simulink model "kirchImplementation"  (R2020b)
settings: Solver=VariableStepAuto  StartTime=0.0  StopTime=Ts  RelTol=1e-3
InitFcn:
  | evalin('base','pixelcontrolbus');
  | 
  | ROWS = 480;
  | COLS = 752;
  | 
  | OFFSET = 2;
  | imagesToRead = 20;
  | Ts = imagesToRead + OFFSET;
  | 
  | inputNums = [1:imagesToRead];
  | 
  | NUM_OF_BITS = 32;
  | MSB = NUM_OF_BITS-1;
  | cap_1 = fixdt(0,NUM_OF_BITS,NUM_OF_BITS-1);
  | cap_2 = fixdt(0,NUM_OF_BITS,NUM_OF_BITS-2);
  | 
  | CORDIC_LUT_DT_1 = fixdt(1, NUM_OF_BITS, NUM_OF_BITS-2);
  | CORDIC_LUT_DT_2 = fixdt(1, NUM_OF_BITS, NUM_OF_BITS-1);
  | CORDIC_LUT_DT_3 = fixdt(1, NUM_OF_BITS, NUM_OF_BITS);
  | CORDIC_LUT_DT_4 = fixdt(1, NUM_OF_BITS, NUM_OF_BITS+1);
  | CORDIC_LUT_DT_5 = fixdt(1, NUM_OF_BITS, NUM_OF_BITS+1);
  | CORDIC_LUT_DT_6 = fixdt(1, NUM_OF_BITS, NUM_OF_BITS+2);
  | CORDIC_LUT_DT_7 = fixdt(1, NUM_OF_BITS, NUM_OF_BITS+3);
  | CORDIC_LUT_DT_8 = fixdt(1, NUM_OF_BITS, NUM_OF_BITS+4);
  | CORDIC_LUT_DT_9 = fixdt(1, NUM_OF_BITS, NUM_OF_BITS+5);
  | CORDIC_LUT_DT_10 = fixdt(1, NUM_OF_BITS, NUM_OF_BITS+6);
  | CORDIC_LUT_DT_11 = fixdt(1, NUM_OF_BITS, NUM_OF_BITS+7);
  | CORDIC_LUT_DT_12 = fixdt(1, NUM_OF_BITS, NUM_OF_BITS+8);
  | 
  | RGB_DT = fixdt(0, 24, 0);
  | GRAY_DT = fixdt(0, 8, 0);
  | THETA_DT = fixdt(1, 16, 13);
  | MAG_DT = fixdt(0, 16, 15);
  | KIRCH_DT = fixdt(0, 12, 0);
  | 
  | OUTPUT_SIZE = RGB_DT.WordLength + ...
  |     GRAY_DT.WordLength + ...
  |     THETA_DT.WordLength + ...
  |     MAG_DT.WordLength + ...
  |     KIRCH_DT.WordLength*4;
  | 
  | RGB_MSB = OUTPUT_SIZE;
  | GRAY_MSB = RGB_MSB - RGB_DT.WordLength;
  | THETA_MSB = GRAY_MSB - GRAY_DT.WordLength;
  | MAG_MSB = THETA_MSB - THETA_DT.WordLength;
  | KIRCH_MSB = MAG_MSB - MAG_DT.WordLength;
StopFcn:
  | for i = inputNums
  | %% Get output data
  | 
  | %raw = out.raw.data(:,:,i+OFFSET);
  | rgb = out.RGB.data(:,:,:,i+OFFSET);
  | gray = out.gray.data(:,:,i+OFFSET);
  | theta = out.theta.data(:,:,i+OFFSET);
  | mag = out.mag.data(:,:,i+OFFSET);
  | kirch_north = uint16(out.kirch_north.data(:,:,i+OFFSET));
  | kirch_northwest = uint16(out.kirch_northwest.data(:,:,i+OFFSET));
  | kirch_west = uint16(out.kirch_west.data(:,:,i+OFFSET));
  | kirch_southwest = uint16(out.kirch_southwest.data(:,:,i+OFFSET));
  | 
  | %% Write out raw data
  | 
  | %writematrix(raw, sprintf("./data/raw%d.csv", i));
  | writematrix(rgb, sprintf("./data/rgb%d.csv", i));
  | writematrix(gray, sprintf("./data/gray%d.csv", i));
  | 
  | writematrix(theta, sprintf("./data/theta%d.csv", i));
  | writematrix(mag, sprintf("./data/mag%d.csv", i));
  | 
  | writematrix(kirch_north, sprintf("./data/kirch_north%d.csv", i));
  | writematrix(kirch_northwest, sprintf("./data/kirch_northwest%d.csv", i));
  | writematrix(kirch_west, sprintf("./data/kirch_west%d.csv", i));
  | writematrix(kirch_southwest, sprintf("./data/kirch_southwest%d.csv", i));
  | end
libraries: hdlsllib x69, visionhdlio x10, simulink x2
(part 1 of 2)
settings Model: Creator=tyson  LastModifiedBy=tyson

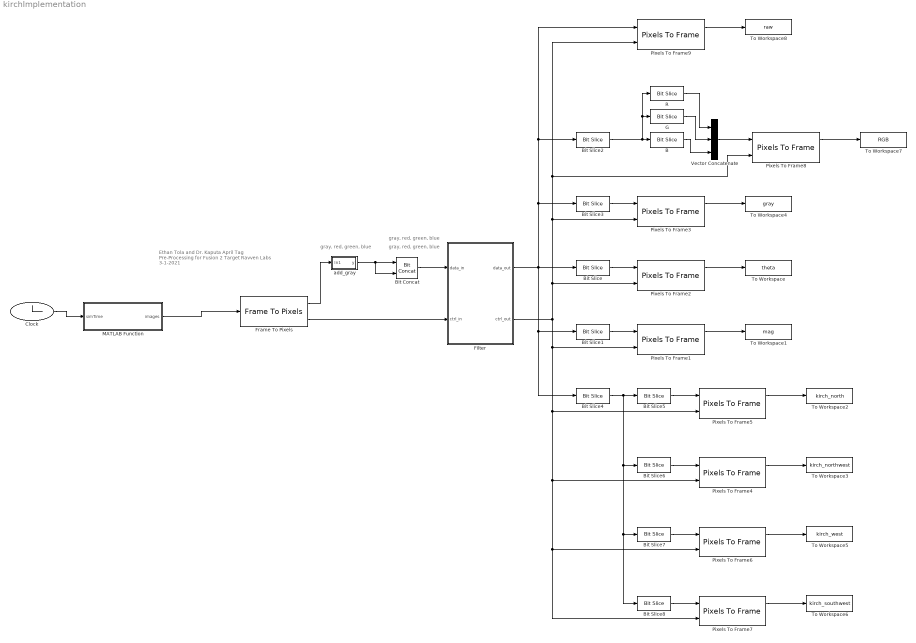
== system kirchImplementation ==
  note: Ethan Tola and Dr. Kaputa
      | April Tag Pre-Processing for Fusion 2 Target
      | Ravven Labs
      | 3-1-2021
  note: gray, red, green, blue
  note: gray, red, green, blue
  note: gray, red, green, blue
  B : hdlsllib/Logic and Bit Operations/Bit Slice  lidx=7  ridx=0
      settings: SourceProductBaseCode=SL
  Bit Concat : hdlsllib/Logic and Bit Operations/Bit Concat  numInputs=2
  Bit Slice : hdlsllib/Logic and Bit Operations/Bit Slice  lidx=THETA_MSB - 1  ridx=THETA_MSB - THETA_DT.WordLength
      settings: SourceProductBaseCode=SL
  Bit Slice1 : hdlsllib/Logic and Bit Operations/Bit Slice  lidx=MAG_MSB - 1  ridx=MAG_MSB - MAG_DT.WordLength
      settings: SourceProductBaseCode=SL
  Bit Slice2 : hdlsllib/Logic and Bit Operations/Bit Slice  lidx=RGB_MSB - 1  ridx=RGB_MSB - RGB_DT.WordLength
      settings: SourceProductBaseCode=SL
  Bit Slice3 : hdlsllib/Logic and Bit Operations/Bit Slice  lidx=GRAY_MSB - 1  ridx=GRAY_MSB - GRAY_DT.WordLength
      settings: SourceProductBaseCode=SL
  Bit Slice4 : hdlsllib/Logic and Bit Operations/Bit Slice  lidx=KIRCH_MSB - 1  ridx=0
      settings: SourceProductBaseCode=SL
  Bit Slice5 : hdlsllib/Logic and Bit Operations/Bit Slice  lidx=KIRCH_MSB - 1  ridx=KIRCH_MSB - KIRCH_DT.WordLength * 1
      settings: SourceProductBaseCode=SL
  Bit Slice6 : hdlsllib/Logic and Bit Operations/Bit Slice  lidx=KIRCH_MSB - (KIRCH_DT.WordLength * 1) - 1  ridx=KIRCH_MSB - KIRCH_DT.WordLength * 2
      settings: SourceProductBaseCode=SL
  Bit Slice7 : hdlsllib/Logic and Bit Operations/Bit Slice  lidx=KIRCH_MSB - (KIRCH_DT.WordLength * 2) - 1  ridx=KIRCH_MSB - KIRCH_DT.WordLength * 3
      settings: SourceProductBaseCode=SL
  Bit Slice8 : hdlsllib/Logic and Bit Operations/Bit Slice  lidx=KIRCH_MSB - (KIRCH_DT.WordLength * 3) - 1  ridx=0
      settings: SourceProductBaseCode=SL
  Clock : Clock
  Filter : Subsystem  TreatAsAtomicUnit=on
  Frame To Pixels : visionhdlio/Frame To Pixels  NumComponents=3  NumPixels=1  VideoFormat=Custom  ActivePixelsPerLine=752  ActiveVideoLines=480  TotalPixelsPerLine=752  TotalVideoLines=480  StartingActiveLine=1  FrontPorch=0  SampleTime=0
      settings: SourceProductName=Vision HDL Toolbox
  G : hdlsllib/Logic and Bit Operations/Bit Slice  lidx=15  ridx=8
      settings: SourceProductBaseCode=SL
  MATLAB Function : MATLAB Function  TreatAsAtomicUnit=on  SystemSampleTime=1
  Pixels To Frame{1..7,9} (8 alike) : visionhdlio/Pixels To Frame  NumComponents=1  NumPixels=1  VideoFormat=Custom  ActivePixelsPerLine=752  ActiveVideoLines=480  TotalPixelsPerLine=752  TotalVideoLines=480
      settings: SourceProductBaseCode=VT
  Pixels To Frame8 : visionhdlio/Pixels To Frame  NumComponents=3  NumPixels=1  VideoFormat=Custom  ActivePixelsPerLine=752  ActiveVideoLines=480  TotalPixelsPerLine=752  TotalVideoLines=480
      settings: SourceProductBaseCode=VT
  R : hdlsllib/Logic and Bit Operations/Bit Slice  lidx=23  ridx=16
      settings: SourceProductBaseCode=SL
  To Workspace : ToWorkspace  VariableName=theta  SaveFormat=Timeseries  SampleTime=-1
  To Workspace1 : ToWorkspace  VariableName=mag  SaveFormat=Timeseries  SampleTime=-1
  To Workspace2 : ToWorkspace  VariableName=kirch_north  SaveFormat=Timeseries  SampleTime=-1
  To Workspace3 : ToWorkspace  VariableName=kirch_northwest  SaveFormat=Timeseries  SampleTime=-1
  To Workspace4 : ToWorkspace  VariableName=gray  SaveFormat=Timeseries  SampleTime=-1
  To Workspace5 : ToWorkspace  VariableName=kirch_west  SaveFormat=Timeseries  SampleTime=-1
  To Workspace6 : ToWorkspace  VariableName=kirch_southwest  SaveFormat=Timeseries  SampleTime=-1
  To Workspace7 : ToWorkspace  VariableName=RGB  SaveFormat=Timeseries  SampleTime=-1
  To Workspace8 : ToWorkspace  VariableName=raw  SaveFormat=Timeseries  SampleTime=-1
  Vector Concatenate : Concatenate  NumInputs=3  Mode=Multidimensional array  ConcatenateDimension=2
  add_gray : Subsystem
  wires:
  Frame To Pixels/1 -> add_gray/1(In1)
  Bit Concat/1 -> Filter/1(data_in)
  Bit Slice1/1 -> Pixels To Frame1/1
  Bit Slice/1 -> Pixels To Frame2/1
  Pixels To Frame2/1 -> To Workspace/1
  Filter/1(data_out) -> Pixels To Frame9/1, Bit Slice2/1, Bit Slice3/1, Bit Slice/1, Bit Slice4/1, Bit Slice1/1
  Pixels To Frame1/1 -> To Workspace1/1
  add_gray/1(y) -> Bit Concat/2, Bit Concat/1
  Filter/2(ctrl_out) -> Pixels To Frame9/2, Pixels To Frame8/2, Pixels To Frame3/2, Pixels To Frame2/2, Pixels To Frame7/2, Pixels To Frame6/2, Pixels To Frame4/2, Pixels To Frame5/2, Pixels To Frame1/2
  Frame To Pixels/2 -> Filter/2(ctrl_in)
  Pixels To Frame7/1 -> To Workspace6/1
  Pixels To Frame5/1 -> To Workspace2/1
  Pixels To Frame4/1 -> To Workspace3/1
  Pixels To Frame6/1 -> To Workspace5/1
  Pixels To Frame3/1 -> To Workspace4/1
  Pixels To Frame8/1 -> To Workspace7/1
  Bit Slice3/1 -> Pixels To Frame3/1
  Bit Slice8/1 -> Pixels To Frame7/1
  Bit Slice7/1 -> Pixels To Frame6/1
  Bit Slice6/1 -> Pixels To Frame4/1
  Bit Slice5/1 -> Pixels To Frame5/1
  Bit Slice4/1 -> Bit Slice8/1, Bit Slice7/1, Bit Slice6/1, Bit Slice5/1
  R/1 -> Vector Concatenate/1
  G/1 -> Vector Concatenate/2
  B/1 -> Vector Concatenate/3
  Bit Slice2/1 -> R/1, G/1, B/1
  Vector Concatenate/1 -> Pixels To Frame8/1
  Pixels To Frame9/1 -> To Workspace8/1
  MATLAB Function/1(images) -> Frame To Pixels/1
  Clock/1 -> MATLAB Function/1(simTime)

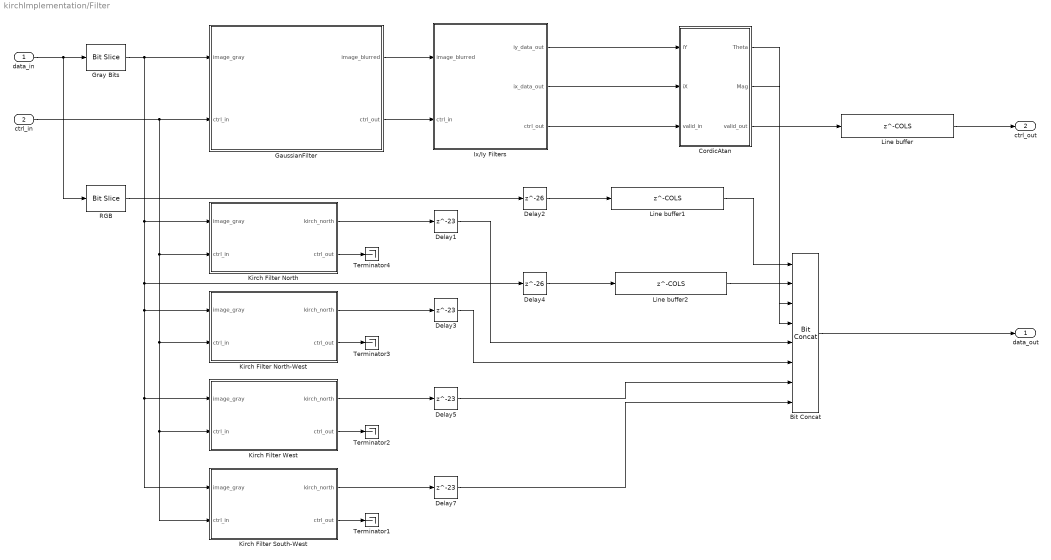
== system kirchImplementation/Filter ==
  data_in : Inport
  ctrl_in : Inport  Port=2
  Bit Concat : hdlsllib/Logic and Bit Operations/Bit Concat  numInputs=8
  CordicAtan : Subsystem
  Delay{1,3,5,7} (4 alike) : Delay  DelayLength=23
  Delay2 : Delay  DelayLength=26
  Delay4 : Delay  DelayLength=26
  GaussianFilter : Subsystem
  Gray Bits : hdlsllib/Logic and Bit Operations/Bit Slice  lidx=31  ridx=24
      settings: SourceProductBaseCode=SL
  Ix/Iy Filters : Subsystem
  Kirch Filter North : Subsystem
  Kirch Filter North-West : Subsystem
  Kirch Filter South-West : Subsystem
  Kirch Filter West : Subsystem
  Line buffer : Delay  DelayLength=COLS  InitialCondition=0
  Line buffer1 : Delay  DelayLength=COLS  InitialCondition=0
  Line buffer2 : Delay  DelayLength=COLS  InitialCondition=0
  RGB : hdlsllib/Logic and Bit Operations/Bit Slice  lidx=23  ridx=0
      settings: SourceProductBaseCode=SL
  Terminator{1..4} (4 alike) : Terminator
  data_out : Outport
  ctrl_out : Outport  Port=2
  wires:
  ctrl_in/1 -> Kirch Filter South-West/2(ctrl_in), Kirch Filter West/2(ctrl_in), Kirch Filter North-West/2(ctrl_in), Kirch Filter North/2(ctrl_in), GaussianFilter/2(ctrl_in)
  Ix/Iy Filters/3(ctrl_out) -> CordicAtan/3(valid_in)
  GaussianFilter/2(ctrl_out) -> Ix/Iy Filters/2(ctrl_in)
  GaussianFilter/1(image_blurred) -> Ix/Iy Filters/1(image_blurred)
  Ix/Iy Filters/2(ix_data_out) -> CordicAtan/2(iX)
  Ix/Iy Filters/1(iy_data_out) -> CordicAtan/1(iY)
  data_in/1 -> RGB/1, Gray Bits/1
  Gray Bits/1 -> Kirch Filter South-West/1(image_gray), Kirch Filter West/1(image_gray), Kirch Filter North-West/1(image_gray), Delay4/1, Kirch Filter North/1(image_gray), GaussianFilter/1(image_gray)
  Kirch Filter North/1(kirch_north) -> Delay1/1
  Kirch Filter North-West/1(kirch_north) -> Delay3/1
  Kirch Filter West/1(kirch_north) -> Delay5/1
  Kirch Filter South-West/1(kirch_north) -> Delay7/1
  Kirch Filter South-West/2(ctrl_out) -> Terminator1/1
  Kirch Filter West/2(ctrl_out) -> Terminator2/1
  Kirch Filter North-West/2(ctrl_out) -> Terminator3/1
  Kirch Filter North/2(ctrl_out) -> Terminator4/1
  Bit Concat/1 -> data_out/1
  RGB/1 -> Delay2/1
  Delay4/1 -> Line buffer2/1
  CordicAtan/3(valid_out) -> Line buffer/1
  Delay2/1 -> Line buffer1/1
  Line buffer/1 -> ctrl_out/1
  Line buffer1/1 -> Bit Concat/1
  Line buffer2/1 -> Bit Concat/2
  CordicAtan/1(Theta) -> Bit Concat/3
  CordicAtan/2(Mag) -> Bit Concat/4
  Delay1/1 -> Bit Concat/5
  Delay3/1 -> Bit Concat/6
  Delay5/1 -> Bit Concat/7
  Delay7/1 -> Bit Concat/8

== system kirchImplementation/add_gray ==
  note: Grayscale = (R * 0.25) + (G * 0.5) + (B * 0.125)
  In1 : Inport
  Bit Concat : hdlsllib/Logic and Bit Operations/Bit Concat  numInputs=4
  Demux : Demux  Outputs=3
  Shift Arithmetic3 : ArithShift  BitShiftNumber=1  BitShiftDirection=Right
  Shift Arithmetic4 : ArithShift  BitShiftNumber=2  BitShiftDirection=Right
  Shift Arithmetic5 : ArithShift  BitShiftNumber=3  BitShiftDirection=Right
  Sum : Sum  Inputs=+++  OutDataTypeStr=uint8
  y : Outport
  wires:
  Bit Concat/1 -> y/1
  In1/1 -> Demux/1
  Demux/2 -> Shift Arithmetic3/1, Bit Concat/3
  Demux/1 -> Shift Arithmetic4/1, Bit Concat/2
  Demux/3 -> Shift Arithmetic5/1, Bit Concat/4
  Sum/1 -> Bit Concat/1
  Shift Arithmetic4/1 -> Sum/1
  Shift Arithmetic3/1 -> Sum/2
  Shift Arithmetic5/1 -> Sum/3

== system kirchImplementation/Filter/CordicAtan ==
  iY : Inport
  iX : Inport  Port=2
  valid_in : Inport  Port=3
  Bus Selector : BusSelector  OutputSignals=valid
  CORDIC Algorithm : Subsystem
  Delay32 : Delay  DelayLength=14
  Theta : Outport
  Mag : Outport  Port=2
  valid_out : Outport  Port=3
  wires:
  Delay32/1 -> valid_out/1
  iY/1 -> CORDIC Algorithm/1(In1)
  iX/1 -> CORDIC Algorithm/2(In2)
  CORDIC Algorithm/1(Out1) -> Theta/1
  CORDIC Algorithm/2(Out2) -> Mag/1
  valid_in/1 -> Delay32/1, Bus Selector/1
  Bus Selector/1 -> CORDIC Algorithm/Enable  "<valid>"

== system kirchImplementation/Filter/GaussianFilter ==
  image_gray : Inport
  ctrl_in : Inport  Port=2
  Bus Selector : BusSelector  OutputSignals=valid
  Constant : Constant  Value=[0.225610111284052,0.548779777431897,0.225610111284052]  OutDataTypeStr=Inherit: Inherit via back propagation  SampleTime=-1
  Constant1 : Constant  Value=[0.225610111284051;0.548779777431897;0.225610111284052]  OutDataTypeStr=Inherit: Inherit via back propagation  SampleTime=-1
  Data Type Duplicate : DataTypeDuplicate  NumInputPorts=3
  Delay : Delay
  Delay1 : Delay  DelayLength=4
  Delay2 : Delay  DelayLength=4
  Normalize : Gain  Gain=1/255  OutDataTypeStr=cap_1
  Symmetric Filter : Subsystem
  image_blurred : Outport
  ctrl_out : Outport  Port=2
  wires:
  ctrl_in/1 -> Bus Selector/1, Delay/1
  Constant/1 -> Data Type Duplicate/1, Symmetric Filter/2(horizontal_coefficients)
  Delay/1 -> Delay1/1
  Bus Selector/1 -> Symmetric Filter/Enable  "<valid>"
  Constant1/1 -> Data Type Duplicate/2, Symmetric Filter/1(verticle_coefficients)
  Delay1/1 -> Delay2/1
  Normalize/1 -> Data Type Duplicate/3, Symmetric Filter/3(data_in)
  image_gray/1 -> Normalize/1
  Delay2/1 -> ctrl_out/1
  Symmetric Filter/1(data_out) -> image_blurred/1

== system kirchImplementation/Filter/Ix//Iy Filters ==
  image_blurred : Inport
  ctrl_in : Inport  Port=2
  Delay1 : Delay
  Ix Filter : Subsystem
  Iy Filter : Subsystem
  iy_data_out : Outport
  ix_data_out : Outport  Port=2
  ctrl_out : Outport  Port=3
  wires:
  Iy Filter/1(data_out) -> iy_data_out/1
  image_blurred/1 -> Iy Filter/1(data_in), Ix Filter/1(data_in)
  Delay1/1 -> ctrl_out/1
  ctrl_in/1 -> Iy Filter/2(ctrl_in), Delay1/1, Ix Filter/2(ctrl_in)
  Ix Filter/1(data_out) -> ix_data_out/1

== system kirchImplementation/Filter/Kirch Filter North ==
  image_gray : Inport
  ctrl_in : Inport  Port=2
  Bus Selector : BusSelector  OutputSignals=valid
  Delay4 : Delay  DelayLength=3
  Kirch Filter : Subsystem
  kirch_north : Outport
  ctrl_out : Outport  Port=2
  wires:
  Delay4/1 -> ctrl_out/1
  ctrl_in/1 -> Bus Selector/1, Delay4/1
  image_gray/1 -> Kirch Filter/1(data_in)
  Kirch Filter/1(Out1) -> kirch_north/1
  Bus Selector/1 -> Kirch Filter/Enable  "<valid>"

== system kirchImplementation/Filter/Kirch Filter North-West ==
  image_gray : Inport
  ctrl_in : Inport  Port=2
  Bus Selector : BusSelector  OutputSignals=valid
  Delay4 : Delay  DelayLength=3
  Kirch Filter : Subsystem
  kirch_north : Outport
  ctrl_out : Outport  Port=2
  wires:
  Delay4/1 -> ctrl_out/1
  ctrl_in/1 -> Delay4/1, Bus Selector/1
  image_gray/1 -> Kirch Filter/1(data_in)
  Kirch Filter/1(Out1) -> kirch_north/1
  Bus Selector/1 -> Kirch Filter/Enable  "<valid>"

== system kirchImplementation/Filter/Kirch Filter South-West ==
  image_gray : Inport
  ctrl_in : Inport  Port=2
  Bus Selector : BusSelector  OutputSignals=valid
  Delay4 : Delay  DelayLength=3
  Subsystem : Subsystem
  kirch_north : Outport
  ctrl_out : Outport  Port=2
  wires:
  Delay4/1 -> ctrl_out/1
  ctrl_in/1 -> Bus Selector/1, Delay4/1
  image_gray/1 -> Subsystem/1(data_in)
  Subsystem/1(Out1) -> kirch_north/1
  Bus Selector/1 -> Subsystem/Enable  "<valid>"

== system kirchImplementation/Filter/Kirch Filter West ==
  image_gray : Inport
  ctrl_in : Inport  Port=2
  Bus Selector : BusSelector  OutputSignals=valid
  Delay4 : Delay  DelayLength=3
  Subsystem : Subsystem
  kirch_north : Outport
  ctrl_out : Outport  Port=2
  wires:
  Delay4/1 -> ctrl_out/1
  ctrl_in/1 -> Bus Selector/1, Delay4/1
  image_gray/1 -> Subsystem/1(data_in)
  Subsystem/1(Out1) -> kirch_north/1
  Bus Selector/1 -> Subsystem/Enable  "<valid>"

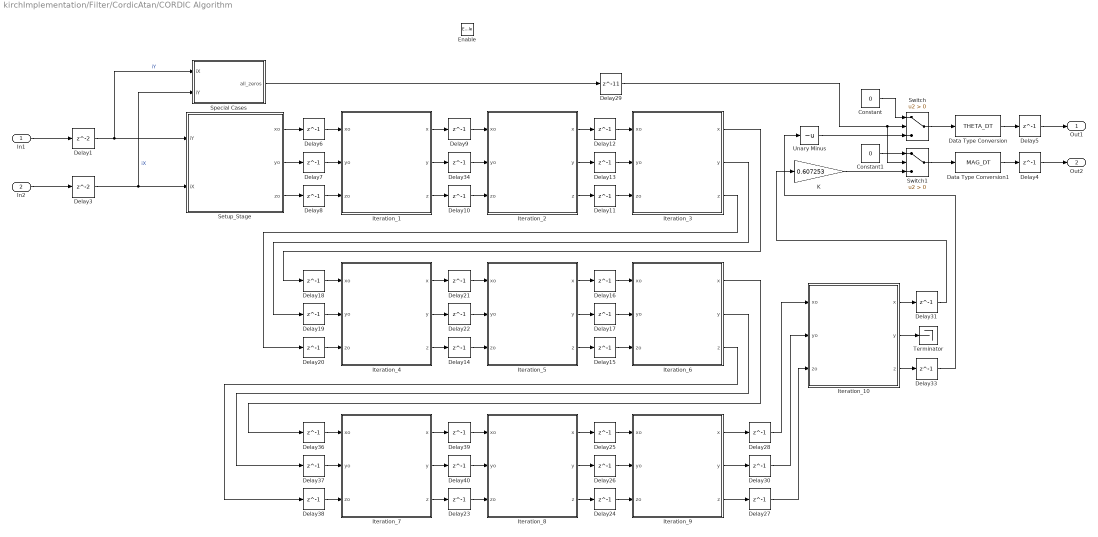
== system kirchImplementation/Filter/CordicAtan/CORDIC Algorithm ==
  In1 : Inport
  In2 : Inport  Port=2
  Enable : EnablePort
  Constant : Constant  Value=0  OutDataTypeStr=Inherit: Inherit via back propagation  SampleTime=-1
  Constant1 : Constant  Value=0  OutDataTypeStr=Inherit: Inherit via back propagation  SampleTime=-1
  Data Type Conversion : DataTypeConversion  OutDataTypeStr=THETA_DT
  Data Type Conversion1 : DataTypeConversion  OutDataTypeStr=MAG_DT
  Delay1 : Delay
  Delay{4..28,30..31,33..34,36..40} (34 alike) : Delay  DelayLength=1
  Delay29 : Delay  DelayLength=11
  Delay3 : Delay
  Iteration_1 : Subsystem
  Iteration_10 : Subsystem
  Iteration_2 : Subsystem
  Iteration_3 : Subsystem
  Iteration_4 : Subsystem
  Iteration_5 : Subsystem
  Iteration_6 : Subsystem
  Iteration_7 : Subsystem
  Iteration_8 : Subsystem
  Iteration_9 : Subsystem
  K : Gain  Gain=0.607253  OutDataTypeStr=fixdt(0,32, 31)
  Setup_Stage : Subsystem
  Special Cases : Subsystem
  Switch : Switch  Criteria=u2 > Threshold
  Switch1 : Switch  Criteria=u2 > Threshold
  Terminator : Terminator
  Unary Minus : UnaryMinus
  Out1 : Outport
  Out2 : Outport  Port=2
  wires:
  Delay12/1 -> Iteration_3/1(xo)
  Iteration_9/1(x) -> Delay28/1
  Delay30/1 -> Iteration_10/2(yo)
  Iteration_6/3(z) -> Delay38/1
  Iteration_1/1(x) -> Delay9/1
  Iteration_3/3(z) -> Delay20/1
  Delay3/1 -> Special Cases/2(iY), Setup_Stage/2(iX)  "iX"
  Iteration_8/2(y) -> Delay26/1
  K/1 -> Switch1/3
  Delay11/1 -> Iteration_3/3(zo)
  Delay13/1 -> Iteration_3/2(yo)
  Delay21/1 -> Iteration_5/1(xo)
  Setup_Stage/2(yo) -> Delay7/1
  Iteration_10/3(z) -> Delay33/1
  Delay29/1 -> Switch1/2, Switch/2
  Delay31/1 -> K/1
  Delay33/1 -> Unary Minus/1
  Delay16/1 -> Iteration_6/1(xo)
  Delay17/1 -> Iteration_6/2(yo)
  Delay9/1 -> Iteration_2/1(xo)
  Iteration_2/3(z) -> Delay11/1
  Delay28/1 -> Iteration_10/1(xo)
  Delay20/1 -> Iteration_4/3(zo)
  Delay22/1 -> Iteration_5/2(yo)
  Delay8/1 -> Iteration_1/3(zo)
  Iteration_3/1(x) -> Delay18/1
  Data Type Conversion1/1 -> Delay4/1
  Iteration_4/3(z) -> Delay14/1
  Delay23/1 -> Iteration_8/3(zo)
  Delay18/1 -> Iteration_4/1(xo)
  Delay40/1 -> Iteration_8/2(yo)
  Iteration_5/2(y) -> Delay17/1
  Iteration_7/2(y) -> Delay40/1
  Setup_Stage/3(zo) -> Delay8/1
  Delay34/1 -> Iteration_2/2(yo)
  Iteration_9/2(y) -> Delay30/1
  Delay25/1 -> Iteration_9/1(xo)
  Iteration_5/1(x) -> Delay16/1
  Iteration_1/3(z) -> Delay10/1
  Delay7/1 -> Iteration_1/2(yo)
  Iteration_7/3(z) -> Delay23/1
  Delay15/1 -> Iteration_6/3(zo)
  Iteration_2/1(x) -> Delay12/1
  Special Cases/1(all_zeros) -> Delay29/1
  Setup_Stage/1(xo) -> Delay6/1
  Delay6/1 -> Iteration_1/1(xo)
  Iteration_4/1(x) -> Delay21/1
  Data Type Conversion/1 -> Delay5/1
  Iteration_3/2(y) -> Delay19/1
  Iteration_4/2(y) -> Delay22/1
  Iteration_6/2(y) -> Delay37/1
  Iteration_9/3(z) -> Delay27/1
  Delay39/1 -> Iteration_8/1(xo)
  Iteration_2/2(y) -> Delay13/1
  Iteration_8/1(x) -> Delay25/1
  Iteration_1/2(y) -> Delay34/1
  Delay10/1 -> Iteration_2/3(zo)
  Iteration_8/3(z) -> Delay24/1
  Delay38/1 -> Iteration_7/3(zo)
  Delay26/1 -> Iteration_9/2(yo)
  Iteration_7/1(x) -> Delay39/1
  Delay19/1 -> Iteration_4/2(yo)
  Iteration_10/2(y) -> Terminator/1
  Iteration_6/1(x) -> Delay36/1
  Delay1/1 -> Special Cases/1(iX), Setup_Stage/1(iY)  "iY"
  Delay36/1 -> Iteration_7/1(xo)
  Iteration_5/3(z) -> Delay15/1
  Delay37/1 -> Iteration_7/2(yo)
  Delay24/1 -> Iteration_9/3(zo)
  Unary Minus/1 -> Switch/3
  Delay27/1 -> Iteration_10/3(zo)
  Constant/1 -> Switch/1
  Delay14/1 -> Iteration_5/3(zo)
  Iteration_10/1(x) -> Delay31/1
  Switch1/1 -> Data Type Conversion1/1
  Switch/1 -> Data Type Conversion/1
  Constant1/1 -> Switch1/1
  In1/1 -> Delay1/1
  In2/1 -> Delay3/1
  Delay5/1 -> Out1/1
  Delay4/1 -> Out2/1

== system kirchImplementation/Filter/GaussianFilter/Symmetric Filter ==
  verticle_coefficients : Inport
  horizontal_coefficients : Inport  Port=2
  data_in : Inport  Port=3
  Enable : EnablePort
  Mux : Mux  Inputs=3
  Row Filter1 : Subsystem
  Row Filter2 : Subsystem
  Row Filter3 : Subsystem
  Verticle Filter : Subsystem
  slicer : Subsystem
  data_out : Outport  InitialOutput=0
  wires:
  Row Filter2/1(data_out) -> Mux/2
  Row Filter3/1(data_out) -> Mux/3
  Row Filter1/1(data_out) -> Mux/1
  slicer/1(Row1) -> Row Filter1/1(data_in)
  data_in/1 -> slicer/1(data_in)
  horizontal_coefficients/1 -> Row Filter3/2(coefficients), Row Filter2/2(coefficients), Row Filter1/2(coefficients)
  slicer/2(Row2) -> Row Filter2/1(data_in)
  slicer/3(Row3) -> Row Filter3/1(data_in)
  Mux/1 -> Verticle Filter/1(data_in)
  Verticle Filter/1(data_out) -> data_out/1
  verticle_coefficients/1 -> Verticle Filter/2(coefficients)

== system kirchImplementation/Filter/Ix//Iy Filters/Ix Filter ==
  data_in : Inport
  ctrl_in : Inport  Port=2
  Bus Selector : BusSelector  OutputSignals=valid
  Filter : Subsystem
  data_out : Outport
  wires:
  ctrl_in/1 -> Bus Selector/1
  data_in/1 -> Filter/1(data_in)
  Filter/1(data_out) -> data_out/1
  Bus Selector/1 -> Filter/Enable  "<valid>"

== system kirchImplementation/Filter/Ix//Iy Filters/Iy Filter ==
  data_in : Inport
  ctrl_in : Inport  Port=2
  Bus Selector : BusSelector  OutputSignals=valid
  Filter : Subsystem
  data_out : Outport
  wires:
  ctrl_in/1 -> Bus Selector/1
  data_in/1 -> Filter/1(data_in)
  Filter/1(data_out) -> data_out/1
  Bus Selector/1 -> Filter/Enable  "<valid>"

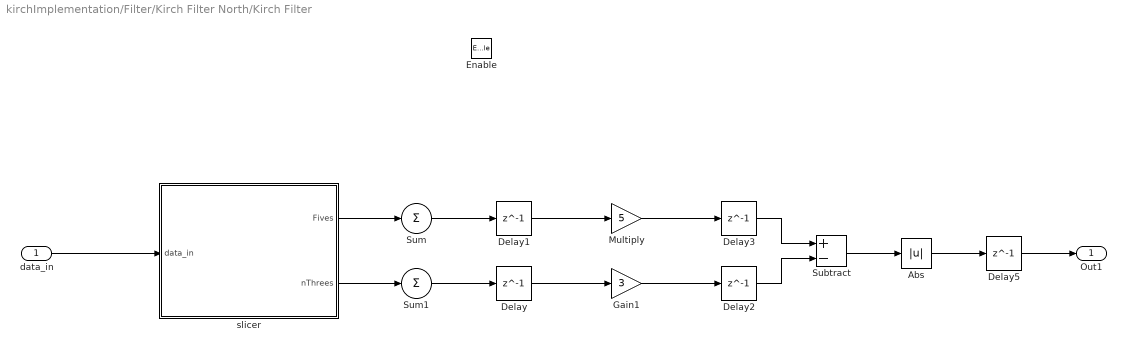
== system kirchImplementation/Filter/Kirch Filter North/Kirch Filter ==
  data_in : Inport
  Enable : EnablePort
  Abs : Abs  OutDataTypeStr=fixdt(0,12,0)
  Delay{,1..3,5} (5 alike) : Delay  DelayLength=1
  Gain1 : Gain  Gain=3  OutDataTypeStr=fixdt(0,13,0)
  Multiply : Gain  Gain=5  OutDataTypeStr=fixdt(0,13,0)
  Subtract : Sum  Inputs=+-  OutDataTypeStr=fixdt(1,13,0)
  Sum : Sum  Inputs=+  OutDataTypeStr=fixdt(0,10,0)
  Sum1 : Sum  Inputs=+  OutDataTypeStr=fixdt(0,11,0)
  slicer : Subsystem
  Out1 : Outport
  wires:
  slicer/2(nThrees) -> Sum1/1
  slicer/1(Fives) -> Sum/1
  Sum/1 -> Delay1/1
  Delay/1 -> Gain1/1
  Delay1/1 -> Multiply/1
  Subtract/1 -> Abs/1
  Sum1/1 -> Delay/1
  Abs/1 -> Delay5/1
  Delay2/1 -> Subtract/2
  Gain1/1 -> Delay2/1
  Delay3/1 -> Subtract/1
  Multiply/1 -> Delay3/1
  data_in/1 -> slicer/1(data_in)
  Delay5/1 -> Out1/1

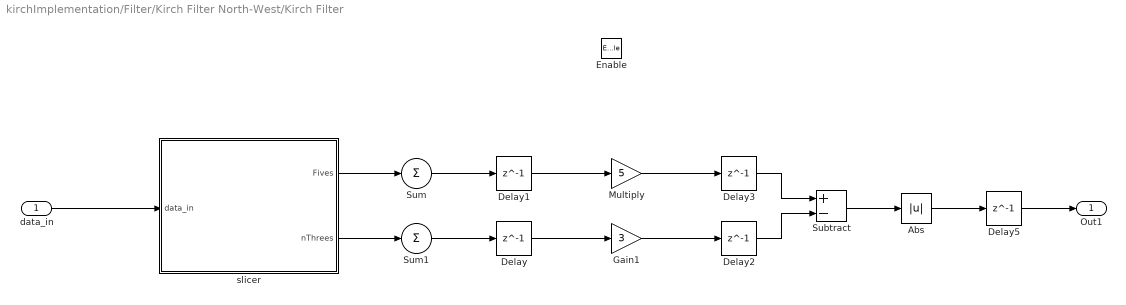
== system kirchImplementation/Filter/Kirch Filter North-West/Kirch Filter ==
  data_in : Inport
  Enable : EnablePort
  Abs : Abs  OutDataTypeStr=fixdt(0,12,0)
  Delay{,1..3,5} (5 alike) : Delay  DelayLength=1
  Gain1 : Gain  Gain=3  OutDataTypeStr=fixdt(0,13,0)
  Multiply : Gain  Gain=5  OutDataTypeStr=fixdt(0,13,0)
  Subtract : Sum  Inputs=+-  OutDataTypeStr=fixdt(1,13,0)
  Sum : Sum  Inputs=+  OutDataTypeStr=fixdt(0,10,0)
  Sum1 : Sum  Inputs=+  OutDataTypeStr=fixdt(0,11,0)
  slicer : Subsystem
  Out1 : Outport
  wires:
  Sum/1 -> Delay1/1
  Subtract/1 -> Abs/1
  Gain1/1 -> Delay2/1
  Multiply/1 -> Delay3/1
  slicer/2(nThrees) -> Sum1/1
  Sum1/1 -> Delay/1
  Delay3/1 -> Subtract/1
  Delay/1 -> Gain1/1
  Delay1/1 -> Multiply/1
  Abs/1 -> Delay5/1
  slicer/1(Fives) -> Sum/1
  Delay2/1 -> Subtract/2
  data_in/1 -> slicer/1(data_in)
  Delay5/1 -> Out1/1

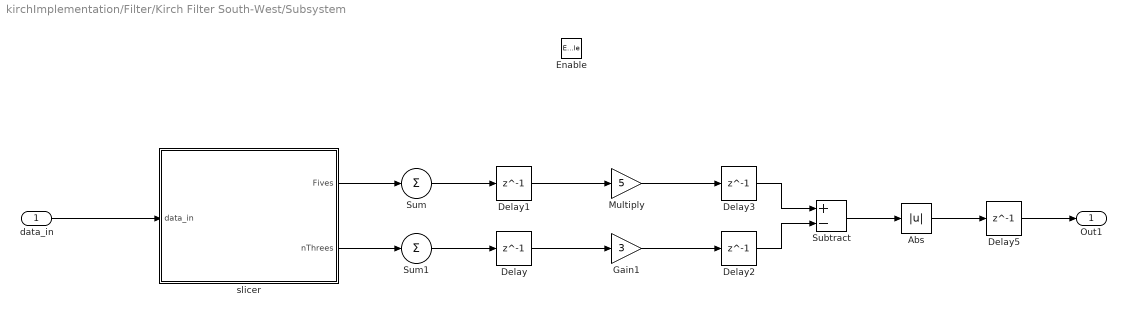
== system kirchImplementation/Filter/Kirch Filter South-West/Subsystem ==
  data_in : Inport
  Enable : EnablePort
  Abs : Abs  OutDataTypeStr=fixdt(0,12,0)
  Delay{,1..3,5} (5 alike) : Delay  DelayLength=1
  Gain1 : Gain  Gain=3  OutDataTypeStr=fixdt(0,13,0)
  Multiply : Gain  Gain=5  OutDataTypeStr=fixdt(0,13,0)
  Subtract : Sum  Inputs=+-  OutDataTypeStr=fixdt(1,13,0)
  Sum : Sum  Inputs=+  OutDataTypeStr=fixdt(0,10,0)
  Sum1 : Sum  Inputs=+  OutDataTypeStr=fixdt(0,11,0)
  slicer : Subsystem
  Out1 : Outport
  wires:
  Delay1/1 -> Multiply/1
  slicer/2(nThrees) -> Sum1/1
  Delay/1 -> Gain1/1
  Gain1/1 -> Delay2/1
  Delay3/1 -> Subtract/1
  Subtract/1 -> Abs/1
  slicer/1(Fives) -> Sum/1
  Multiply/1 -> Delay3/1
  Abs/1 -> Delay5/1
  Delay5/1 -> Out1/1
  Delay2/1 -> Subtract/2
  Sum/1 -> Delay1/1
  Sum1/1 -> Delay/1
  data_in/1 -> slicer/1(data_in)

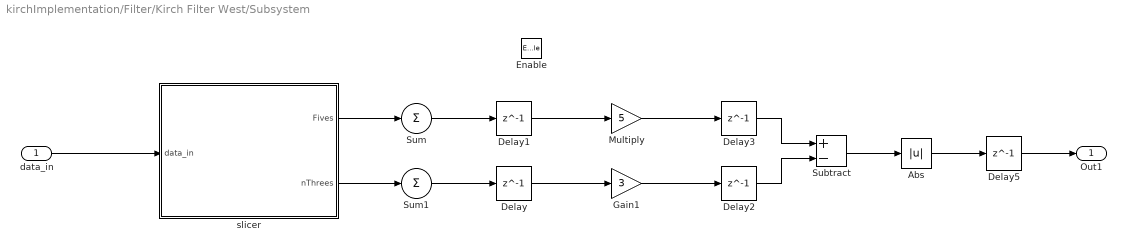
== system kirchImplementation/Filter/Kirch Filter West/Subsystem ==
  data_in : Inport
  Enable : EnablePort
  Abs : Abs  OutDataTypeStr=fixdt(0,12,0)
  Delay{,1..3,5} (5 alike) : Delay  DelayLength=1
  Gain1 : Gain  Gain=3  OutDataTypeStr=fixdt(0,13,0)
  Multiply : Gain  Gain=5  OutDataTypeStr=fixdt(0,13,0)
  Subtract : Sum  Inputs=+-  OutDataTypeStr=fixdt(1,13,0)
  Sum : Sum  Inputs=+  OutDataTypeStr=fixdt(0,10,0)
  Sum1 : Sum  Inputs=+  OutDataTypeStr=fixdt(0,11,0)
  slicer : Subsystem
  Out1 : Outport
  wires:
  Subtract/1 -> Abs/1
  Abs/1 -> Delay5/1
  Delay2/1 -> Subtract/2
  Multiply/1 -> Delay3/1
  Delay3/1 -> Subtract/1
  Delay1/1 -> Multiply/1
  slicer/1(Fives) -> Sum/1
  Delay/1 -> Gain1/1
  Sum1/1 -> Delay/1
  slicer/2(nThrees) -> Sum1/1
  Sum/1 -> Delay1/1
  Delay5/1 -> Out1/1
  Gain1/1 -> Delay2/1
  data_in/1 -> slicer/1(data_in)

== system kirchImplementation/Filter/CordicAtan/CORDIC Algorithm/Iteration_1 ==
  xo : Inport
  yo : Inport  Port=2
  zo : Inport  Port=3
  Add : Sum
  Add1 : Sum  OutDataTypeStr=fixdt(1,NUM_OF_BITS, NUM_OF_BITS-3)
  Add2 : Sum
  cordicLut_3 : Constant  Value=0.463647609000806  OutDataTypeStr=CORDIC_LUT_DT_3  SampleTime=-1
  n_zsign : Subsystem
  n_zsign1 : Subsystem
  zsign : Subsystem
  x : Outport
  y : Outport  Port=2
  z : Outport  Port=3
  wires:
  Add/1 -> z/1
  cordicLut_3/1 -> n_zsign1/2(base)
  zo/1 -> Add/2
  n_zsign1/1(out) -> Add/1
  yo/1 -> zsign/2(base), zsign/1(signof), n_zsign/1(signof), Add2/2
  zsign/1(out) -> Add1/2  "xo"
  xo/1 -> n_zsign/2(base), Add1/1
  Add1/1 -> x/1
  n_zsign/1(out) -> Add2/1
  Add2/1 -> n_zsign1/1(signof), y/1

== system kirchImplementation/Filter/CordicAtan/CORDIC Algorithm/Iteration_10 ==
  xo : Inport
  yo : Inport  Port=2
  zo : Inport  Port=3
  Add : Sum
  X_Logic : Subsystem
  Y_Logic : Subsystem
  cordicLut_12 : Constant  Value=0.000976562189559320  OutDataTypeStr=CORDIC_LUT_DT_12  SampleTime=-1
  n_zsign : Subsystem
  x : Outport
  y : Outport  Port=2
  z : Outport  Port=3
  wires:
  Add/1 -> z/1
  cordicLut_12/1 -> n_zsign/2(base)
  zo/1 -> Add/2
  n_zsign/1(out) -> Add/1
  yo/1 -> Y_Logic/2(yo), X_Logic/2(yo)
  xo/1 -> Y_Logic/1(xo), X_Logic/1(xo)
  X_Logic/1(x) -> x/1
  Y_Logic/1(y) -> n_zsign/1(signof), y/1

== system kirchImplementation/Filter/CordicAtan/CORDIC Algorithm/Iteration_2 ==
  xo : Inport
  yo : Inport  Port=2
  zo : Inport  Port=3
  Add : Sum
  X_Logic : Subsystem
  Y_Logic : Subsystem
  cordicLut_4 : Constant  Value=0.244978663126864  OutDataTypeStr=CORDIC_LUT_DT_4  SampleTime=-1
  n_zsign : Subsystem
  x : Outport
  y : Outport  Port=2
  z : Outport  Port=3
  wires:
  Add/1 -> z/1
  cordicLut_4/1 -> n_zsign/2(base)
  zo/1 -> Add/2
  n_zsign/1(out) -> Add/1
  yo/1 -> Y_Logic/2(yo), X_Logic/2(yo)
  xo/1 -> Y_Logic/1(xo), X_Logic/1(xo)
  X_Logic/1(x) -> x/1
  Y_Logic/1(y) -> n_zsign/1(signof), y/1

== system kirchImplementation/Filter/CordicAtan/CORDIC Algorithm/Iteration_3 ==
  xo : Inport
  yo : Inport  Port=2
  zo : Inport  Port=3
  Add : Sum
  X_Logic : Subsystem
  Y_Logic : Subsystem
  cordicLut_5 : Constant  Value=0.124354994546761  OutDataTypeStr=CORDIC_LUT_DT_5  SampleTime=-1
  n_zsign : Subsystem
  x : Outport
  y : Outport  Port=2
  z : Outport  Port=3
  wires:
  Add/1 -> z/1
  cordicLut_5/1 -> n_zsign/2(base)
  zo/1 -> Add/2
  n_zsign/1(out) -> Add/1
  yo/1 -> Y_Logic/2(yo), X_Logic/2(yo)
  xo/1 -> Y_Logic/1(xo), X_Logic/1(xo)
  X_Logic/1(x) -> x/1
  Y_Logic/1(y) -> n_zsign/1(signof), y/1

== system kirchImplementation/Filter/CordicAtan/CORDIC Algorithm/Iteration_4 ==
  xo : Inport
  yo : Inport  Port=2
  zo : Inport  Port=3
  Add : Sum
  X_Logic : Subsystem
  Y_Logic : Subsystem
  cordicLut_6 : Constant  Value=0.0624188099959574  OutDataTypeStr=CORDIC_LUT_DT_6  SampleTime=-1
  n_zsign : Subsystem
  x : Outport
  y : Outport  Port=2
  z : Outport  Port=3
  wires:
  Add/1 -> z/1
  cordicLut_6/1 -> n_zsign/2(base)
  zo/1 -> Add/2
  n_zsign/1(out) -> Add/1
  yo/1 -> Y_Logic/2(yo), X_Logic/2(yo)
  xo/1 -> Y_Logic/1(xo), X_Logic/1(xo)
  X_Logic/1(x) -> x/1
  Y_Logic/1(y) -> n_zsign/1(signof), y/1

== system kirchImplementation/Filter/CordicAtan/CORDIC Algorithm/Iteration_5 ==
  xo : Inport
  yo : Inport  Port=2
  zo : Inport  Port=3
  Add : Sum
  X_Logic : Subsystem
  Y_Logic : Subsystem
  cordicLut_7 : Constant  Value=0.0312398334302683  OutDataTypeStr=CORDIC_LUT_DT_7  SampleTime=-1
  n_zsign : Subsystem
  x : Outport
  y : Outport  Port=2
  z : Outport  Port=3
  wires:
  Add/1 -> z/1
  cordicLut_7/1 -> n_zsign/2(base)
  zo/1 -> Add/2
  n_zsign/1(out) -> Add/1
  yo/1 -> Y_Logic/2(yo), X_Logic/2(yo)
  xo/1 -> Y_Logic/1(xo), X_Logic/1(xo)
  X_Logic/1(x) -> x/1
  Y_Logic/1(y) -> n_zsign/1(signof), y/1

== system kirchImplementation/Filter/CordicAtan/CORDIC Algorithm/Iteration_6 ==
  xo : Inport
  yo : Inport  Port=2
  zo : Inport  Port=3
  Add : Sum
  X_Logic : Subsystem
  Y_Logic : Subsystem
  cordicLut_8 : Constant  Value=0.0156237286204768  OutDataTypeStr=CORDIC_LUT_DT_8  SampleTime=-1
  n_zsign : Subsystem
  x : Outport
  y : Outport  Port=2
  z : Outport  Port=3
  wires:
  Add/1 -> z/1
  cordicLut_8/1 -> n_zsign/2(base)
  zo/1 -> Add/2
  n_zsign/1(out) -> Add/1
  yo/1 -> Y_Logic/2(yo), X_Logic/2(yo)
  xo/1 -> Y_Logic/1(xo), X_Logic/1(xo)
  X_Logic/1(x) -> x/1
  Y_Logic/1(y) -> n_zsign/1(signof), y/1

== system kirchImplementation/Filter/CordicAtan/CORDIC Algorithm/Iteration_7 ==
  xo : Inport
  yo : Inport  Port=2
  zo : Inport  Port=3
  Add : Sum
  X_Logic : Subsystem
  Y_Logic : Subsystem
  cordicLut_9 : Constant  Value=0.00781234106010111  OutDataTypeStr=CORDIC_LUT_DT_9  SampleTime=-1
  n_zsign : Subsystem
  x : Outport
  y : Outport  Port=2
  z : Outport  Port=3
  wires:
  Add/1 -> z/1
  cordicLut_9/1 -> n_zsign/2(base)
  zo/1 -> Add/2
  n_zsign/1(out) -> Add/1
  yo/1 -> Y_Logic/2(yo), X_Logic/2(yo)
  xo/1 -> Y_Logic/1(xo), X_Logic/1(xo)
  X_Logic/1(x) -> x/1
  Y_Logic/1(y) -> n_zsign/1(signof), y/1

== system kirchImplementation/Filter/CordicAtan/CORDIC Algorithm/Iteration_8 ==
  xo : Inport
  yo : Inport  Port=2
  zo : Inport  Port=3
  Add : Sum
  X_Logic : Subsystem
  Y_Logic : Subsystem
  cordicLut_10 : Constant  Value=0.00390623013196697  OutDataTypeStr=CORDIC_LUT_DT_10  SampleTime=-1
  n_zsign : Subsystem
  x : Outport
  y : Outport  Port=2
  z : Outport  Port=3
  wires:
  Add/1 -> z/1
  cordicLut_10/1 -> n_zsign/2(base)
  zo/1 -> Add/2
  n_zsign/1(out) -> Add/1
  yo/1 -> Y_Logic/2(yo), X_Logic/2(yo)
  xo/1 -> Y_Logic/1(xo), X_Logic/1(xo)
  X_Logic/1(x) -> x/1
  Y_Logic/1(y) -> n_zsign/1(signof), y/1

== system kirchImplementation/Filter/CordicAtan/CORDIC Algorithm/Iteration_9 ==
  xo : Inport
  yo : Inport  Port=2
  zo : Inport  Port=3
  Add : Sum
  X_Logic : Subsystem
  Y_Logic : Subsystem
  cordicLut_11 : Constant  Value=0.00195312251647882  OutDataTypeStr=CORDIC_LUT_DT_11  SampleTime=-1
  n_zsign : Subsystem
  x : Outport
  y : Outport  Port=2
  z : Outport  Port=3
  wires:
  Add/1 -> z/1
  cordicLut_11/1 -> n_zsign/2(base)
  zo/1 -> Add/2
  n_zsign/1(out) -> Add/1
  yo/1 -> Y_Logic/2(yo), X_Logic/2(yo)
  xo/1 -> Y_Logic/1(xo), X_Logic/1(xo)
  X_Logic/1(x) -> x/1
  Y_Logic/1(y) -> n_zsign/1(signof), y/1

== system kirchImplementation/Filter/CordicAtan/CORDIC Algorithm/Setup_Stage ==
  iY : Inport
  iX : Inport  Port=2
  Add : Sum  OutDataTypeStr=fixdt(1,NUM_OF_BITS,NUM_OF_BITS-3)
  cordicLut_1 : Constant  Value=1.57079632679490  OutDataTypeStr=CORDIC_LUT_DT_1  SampleTime=-1
  cordicLut_2 : Constant  Value=0.785398163397448  OutDataTypeStr=CORDIC_LUT_DT_2  SampleTime=-1
  n_zsign : Subsystem
  n_zsign1 : Subsystem
  n_zsign2 : Subsystem
  zsign : Subsystem
  xo : Outport
  yo : Outport  Port=2
  zo : Outport  Port=3
  wires:
  cordicLut_1/1 -> n_zsign1/2(base)
  iY/1 -> zsign/2(base), n_zsign1/1(signof), n_zsign/1(signof), zsign/1(signof)
  n_zsign/1(out) -> n_zsign2/1(signof), yo/1  "yo"
  n_zsign1/1(out) -> Add/1  "zo"
  cordicLut_2/1 -> n_zsign2/2(base)
  iX/1 -> n_zsign/2(base)
  n_zsign2/1(out) -> Add/2
  Add/1 -> zo/1  "zo"
  zsign/1(out) -> xo/1  "xo"

== system kirchImplementation/Filter/CordicAtan/CORDIC Algorithm/Special Cases ==
  iX : Inport
  iY : Inport  Port=2
  Compare To Zero : simulink/Logic and Bit Operations/Compare To Zero  relop===  OutDataTypeStr=boolean
  Compare To Zero1 : simulink/Logic and Bit Operations/Compare To Zero  relop===  OutDataTypeStr=boolean
  Logical Operator : Logic  AllPortsSameDT=off  OutDataTypeStr=boolean
  all_zeros : Outport
  wires:
  Compare To Zero1/1 -> Logical Operator/2
  Logical Operator/1 -> all_zeros/1
  iY/1 -> Compare To Zero1/1
  Compare To Zero/1 -> Logical Operator/1
  iX/1 -> Compare To Zero/1

== system kirchImplementation/Filter/GaussianFilter/Symmetric Filter/Row Filter1 ==
  data_in : Inport
  coefficients : Inport  Port=2
  Delay1 : Delay
  Delay2 : Delay
  Demux : Demux  Outputs=[2, 1]
  Product : Product  OutDataTypeStr=cap_1
  Sum : Sum  Inputs=1  AccumDataTypeStr=cap_1  OutDataTypeStr=cap_1
  Symmetry : Subsystem
  Terminator : Terminator
  data_out : Outport
  wires:
  Product/1 -> Delay1/1
  Symmetry/1(data_out) -> Product/2
  Delay1/1 -> Sum/1
  Delay2/1 -> data_out/1
  Sum/1 -> Delay2/1
  data_in/1 -> Symmetry/1(data_in)
  coefficients/1 -> Demux/1
  Demux/1 -> Product/1
  Demux/2 -> Terminator/1

== system kirchImplementation/Filter/GaussianFilter/Symmetric Filter/Row Filter2 ==
  data_in : Inport
  coefficients : Inport  Port=2
  Delay1 : Delay
  Delay2 : Delay
  Demux : Demux  Outputs=[2, 1]
  Product : Product  OutDataTypeStr=cap_1
  Sum : Sum  Inputs=1  AccumDataTypeStr=cap_1  OutDataTypeStr=cap_1
  Symmetry : Subsystem
  Terminator : Terminator
  data_out : Outport
  wires:
  Product/1 -> Delay1/1
  Symmetry/1(data_out) -> Product/2
  Delay1/1 -> Sum/1
  Delay2/1 -> data_out/1
  Sum/1 -> Delay2/1
  data_in/1 -> Symmetry/1(data_in)
  coefficients/1 -> Demux/1
  Demux/1 -> Product/1
  Demux/2 -> Terminator/1

== system kirchImplementation/Filter/GaussianFilter/Symmetric Filter/Row Filter3 ==
  data_in : Inport
  coefficients : Inport  Port=2
  Delay1 : Delay
  Delay2 : Delay
  Demux : Demux  Outputs=[2, 1]
  Product : Product  OutDataTypeStr=cap_1
  Sum : Sum  Inputs=1  AccumDataTypeStr=cap_1  OutDataTypeStr=cap_1
  Symmetry : Subsystem
  Terminator : Terminator
  data_out : Outport
  wires:
  Product/1 -> Delay1/1
  Symmetry/1(data_out) -> Product/2
  Delay1/1 -> Sum/1
  Delay2/1 -> data_out/1
  Sum/1 -> Delay2/1
  data_in/1 -> Symmetry/1(data_in)
  coefficients/1 -> Demux/1
  Demux/1 -> Product/1
  Demux/2 -> Terminator/1

== system kirchImplementation/Filter/GaussianFilter/Symmetric Filter/Verticle Filter ==
  data_in : Inport
  coefficients : Inport  Port=2
  Delay1 : Delay
  Delay2 : Delay
  Demux : Demux  Outputs=[2, 1]
  Product : Product  OutDataTypeStr=cap_1
  Sum : Sum  Inputs=1  AccumDataTypeStr=cap_1  OutDataTypeStr=cap_1
  Symmetry : Subsystem
  Terminator : Terminator
  data_out : Outport
  wires:
  Product/1 -> Delay1/1
  Symmetry/1(data_out) -> Product/2
  Delay1/1 -> Sum/1
  Delay2/1 -> data_out/1
  Sum/1 -> Delay2/1
  data_in/1 -> Symmetry/1(data_in)
  coefficients/1 -> Demux/1
  Demux/1 -> Product/1
  Demux/2 -> Terminator/1

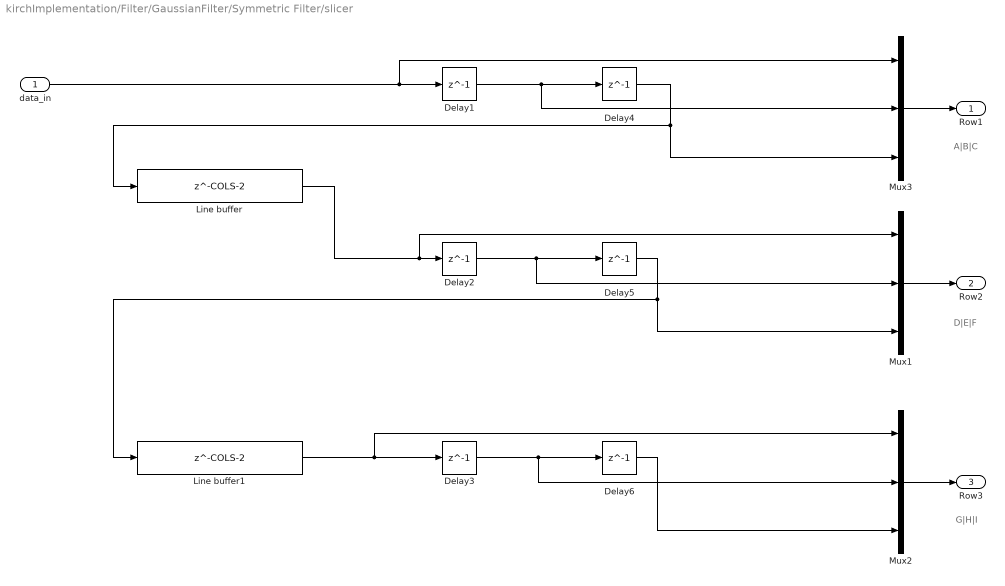
== system kirchImplementation/Filter/GaussianFilter/Symmetric Filter/slicer ==
  note: A|B|C
  note: D|E|F
  note: G|H|I
  data_in : Inport
  Delay{1..6} (6 alike) : Delay  DelayLength=1  InitialCondition=0
  Line buffer : Delay  DelayLength=COLS-2  InitialCondition=0
  Line buffer1 : Delay  DelayLength=COLS-2  InitialCondition=0
  Mux1 : Mux  Inputs=3
  Mux2 : Mux  Inputs=3
  Mux3 : Mux  Inputs=3
  Row1 : Outport  VectorParamsAs1DForOutWhenUnconnected=off
  Row2 : Outport  Port=2  VectorParamsAs1DForOutWhenUnconnected=off
  Row3 : Outport  Port=3  VectorParamsAs1DForOutWhenUnconnected=off
  wires:
  Delay4/1 -> Mux3/3, Line buffer/1
  data_in/1 -> Mux3/1, Delay1/1
  Delay1/1 -> Mux3/2, Delay4/1
  Delay3/1 -> Mux2/2, Delay6/1
  Delay5/1 -> Mux1/3, Line buffer1/1
  Delay6/1 -> Mux2/3
  Line buffer/1 -> Mux1/1, Delay2/1
  Line buffer1/1 -> Mux2/1, Delay3/1
  Delay2/1 -> Mux1/2, Delay5/1
  Mux1/1 -> Row2/1
  Mux2/1 -> Row3/1
  Mux3/1 -> Row1/1

== system kirchImplementation/Filter/Ix//Iy Filters/Ix Filter/Filter ==
  data_in : Inport
  Enable : EnablePort
  Delay : Delay
  Demux : Demux  Outputs=3
  Sum3 : Sum  Inputs=|+-  AccumDataTypeStr=fixdt(1,32,30)  OutDataTypeStr=fixdt(1,32,30)
  Terminator : Terminator
  Terminator1 : Terminator
  Terminator2 : Terminator
  slicer : Subsystem
  data_out : Outport  InitialOutput=0
  wires:
  data_in/1 -> slicer/1(data_in)
  slicer/1(Row1) -> Terminator/1
  slicer/3(Row3) -> Terminator1/1
  slicer/2(Row2) -> Demux/1
  Demux/1 -> Sum3/1
  Demux/3 -> Sum3/2
  Demux/2 -> Terminator2/1
  Delay/1 -> data_out/1
  Sum3/1 -> Delay/1

== system kirchImplementation/Filter/Ix//Iy Filters/Iy Filter/Filter ==
  data_in : Inport
  Enable : EnablePort
  Delay2 : Delay
  Demux : Demux  Outputs=3
  Demux1 : Demux  Outputs=3
  Sum : Sum  Inputs=|+-  AccumDataTypeStr=fixdt(1,32,30)  OutDataTypeStr=fixdt(1,32,30)
  Terminator{,1..4} (5 alike) : Terminator
  slicer : Subsystem
  data_out : Outport  InitialOutput=0
  wires:
  slicer/1(Row1) -> Demux/1
  data_in/1 -> slicer/1(data_in)
  slicer/2(Row2) -> Terminator/1
  slicer/3(Row3) -> Demux1/1
  Demux/1 -> Terminator1/1
  Demux/3 -> Terminator2/1
  Demux/2 -> Sum/1
  Demux1/1 -> Terminator3/1
  Demux1/2 -> Sum/2
  Demux1/3 -> Terminator4/1
  Sum/1 -> Delay2/1
  Delay2/1 -> data_out/1

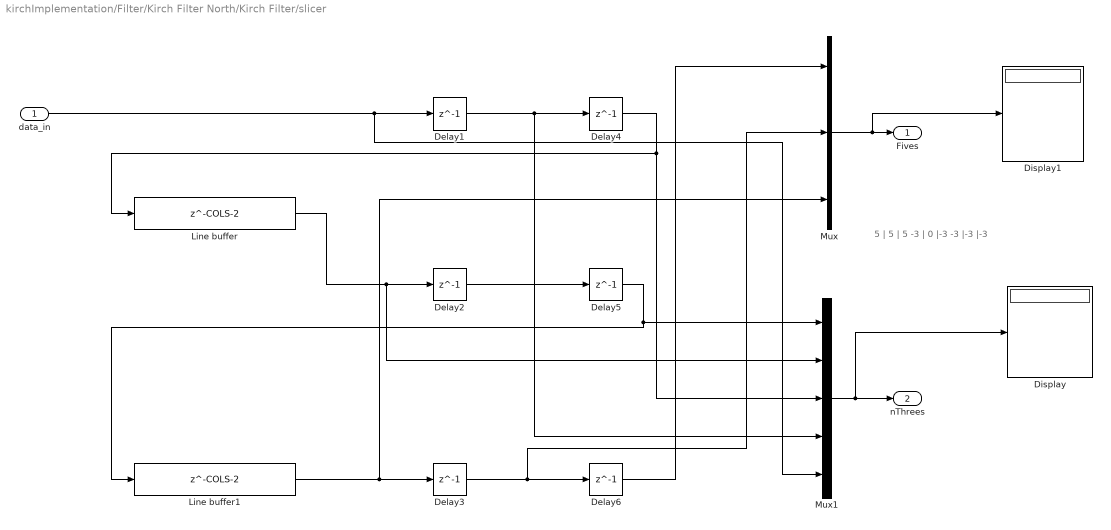
== system kirchImplementation/Filter/Kirch Filter North/Kirch Filter/slicer ==
  note: 5 | 5 | 5
      | -3 | 0 |-3
      | -3 |-3 |-3
  data_in : Inport
  Delay{1..6} (6 alike) : Delay  DelayLength=1  InitialCondition=0
  Display : Display
  Display1 : Display
  Line buffer : Delay  DelayLength=COLS-2  InitialCondition=0
  Line buffer1 : Delay  DelayLength=COLS-2  InitialCondition=0
  Mux : Mux  Inputs=3
  Mux1 : Mux  Inputs=5
  Fives : Outport
  nThrees : Outport  Port=2
  wires:
  Delay4/1 -> Mux1/3, Line buffer/1
  data_in/1 -> Mux1/5, Delay1/1
  Delay1/1 -> Mux1/4, Delay4/1
  Delay3/1 -> Mux/2, Delay6/1
  Delay5/1 -> Line buffer1/1, Mux1/1
  Line buffer/1 -> Mux1/2, Delay2/1
  Line buffer1/1 -> Mux/3, Delay3/1
  Delay2/1 -> Delay5/1
  Mux/1 -> Display1/1, Fives/1
  Mux1/1 -> Display/1, nThrees/1
  Delay6/1 -> Mux/1

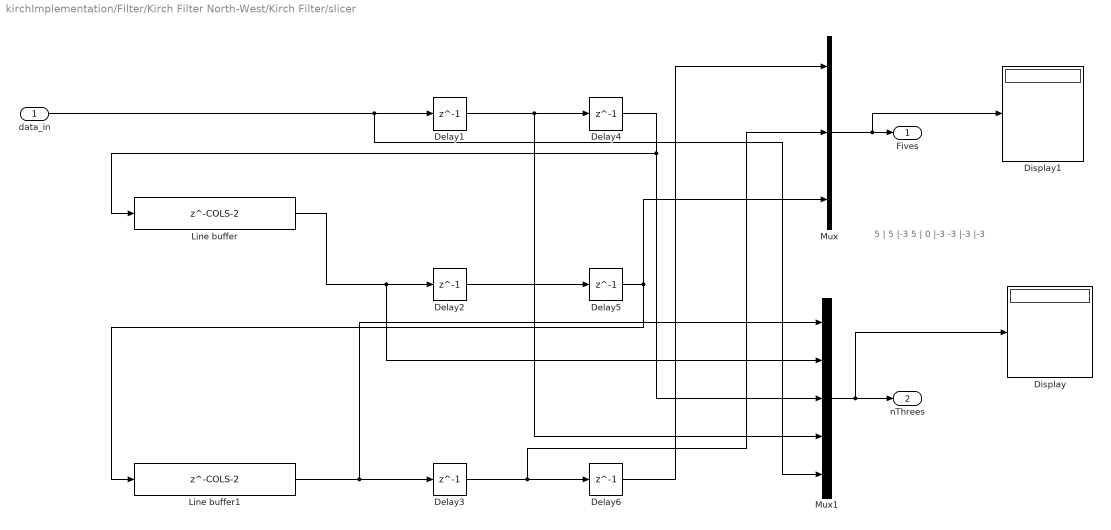
== system kirchImplementation/Filter/Kirch Filter North-West/Kirch Filter/slicer ==
  note: 5 | 5 |-3
      | 5 | 0 |-3
      | -3 |-3 |-3
  data_in : Inport
  Delay{1..6} (6 alike) : Delay  DelayLength=1  InitialCondition=0
  Display : Display
  Display1 : Display
  Line buffer : Delay  DelayLength=COLS-2  InitialCondition=0
  Line buffer1 : Delay  DelayLength=COLS-2  InitialCondition=0
  Mux : Mux  Inputs=3
  Mux1 : Mux  Inputs=5
  Fives : Outport
  nThrees : Outport  Port=2
  wires:
  Delay4/1 -> Mux1/3, Line buffer/1
  data_in/1 -> Mux1/5, Delay1/1
  Delay1/1 -> Mux1/4, Delay4/1
  Delay3/1 -> Mux/2, Delay6/1
  Delay5/1 -> Line buffer1/1, Mux/3
  Line buffer/1 -> Mux1/2, Delay2/1
  Line buffer1/1 -> Delay3/1, Mux1/1
  Delay2/1 -> Delay5/1
  Mux/1 -> Display1/1, Fives/1
  Mux1/1 -> Display/1, nThrees/1
  Delay6/1 -> Mux/1

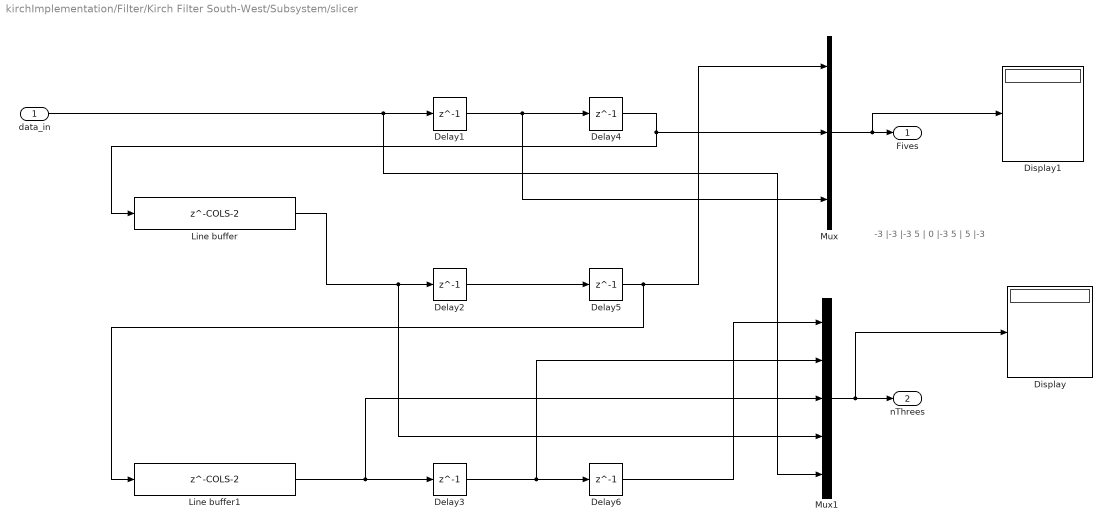
== system kirchImplementation/Filter/Kirch Filter South-West/Subsystem/slicer ==
  note: -3 |-3 |-3
      | 5 | 0 |-3
      | 5 | 5 |-3
  data_in : Inport
  Delay{1..6} (6 alike) : Delay  DelayLength=1  InitialCondition=0
  Display : Display
  Display1 : Display
  Line buffer : Delay  DelayLength=COLS-2  InitialCondition=0
  Line buffer1 : Delay  DelayLength=COLS-2  InitialCondition=0
  Mux : Mux  Inputs=3
  Mux1 : Mux  Inputs=5
  Fives : Outport
  nThrees : Outport  Port=2
  wires:
  Delay4/1 -> Line buffer/1, Mux/2
  data_in/1 -> Mux1/5, Delay1/1
  Delay1/1 -> Mux/3, Delay4/1
  Delay3/1 -> Mux1/2, Delay6/1
  Delay5/1 -> Line buffer1/1, Mux/1
  Line buffer/1 -> Mux1/4, Delay2/1
  Line buffer1/1 -> Mux1/3, Delay3/1
  Delay2/1 -> Delay5/1
  Mux/1 -> Display1/1, Fives/1
  Mux1/1 -> Display/1, nThrees/1
  Delay6/1 -> Mux1/1

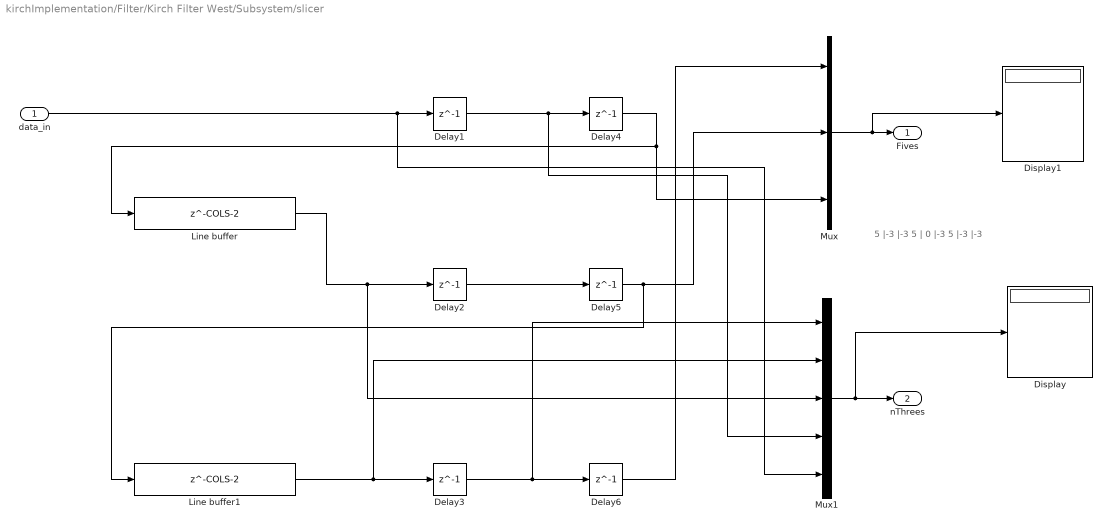
== system kirchImplementation/Filter/Kirch Filter West/Subsystem/slicer ==
  note: 5 |-3 |-3
      | 5 | 0 |-3
      | 5 |-3 |-3
  data_in : Inport
  Delay{1..6} (6 alike) : Delay  DelayLength=1  InitialCondition=0
  Display : Display
  Display1 : Display
  Line buffer : Delay  DelayLength=COLS-2  InitialCondition=0
  Line buffer1 : Delay  DelayLength=COLS-2  InitialCondition=0
  Mux : Mux  Inputs=3
  Mux1 : Mux  Inputs=5
  Fives : Outport
  nThrees : Outport  Port=2
  wires:
  Delay4/1 -> Mux/3, Line buffer/1
  data_in/1 -> Mux1/5, Delay1/1
  Delay1/1 -> Mux1/4, Delay4/1
  Delay3/1 -> Mux1/1, Delay6/1
  Delay5/1 -> Mux/2, Line buffer1/1
  Line buffer/1 -> Mux1/3, Delay2/1
  Line buffer1/1 -> Mux1/2, Delay3/1
  Delay2/1 -> Delay5/1
  Mux/1 -> Display1/1, Fives/1
  Mux1/1 -> Display/1, nThrees/1
  Delay6/1 -> Mux/1

== system kirchImplementation/Filter/CordicAtan/CORDIC Algorithm/Iteration_1/n_zsign ==
  signof : Inport
  base : Inport  Port=2
  Bit Slice : hdlsllib/Logic and Bit Operations/Bit Slice  lidx=MSB  ridx=MSB
      settings: SourceProductBaseCode=SL
  Switch : Switch  Criteria=u2 > Threshold
  Unary Minus : UnaryMinus
  out : Outport
  wires:
  Bit Slice/1 -> Switch/2
  signof/1 -> Bit Slice/1
  base/1 -> Switch/1, Unary Minus/1
  Switch/1 -> out/1
  Unary Minus/1 -> Switch/3

== system kirchImplementation/Filter/CordicAtan/CORDIC Algorithm/Iteration_1/n_zsign1 ==
  signof : Inport
  base : Inport  Port=2
  Bit Slice : hdlsllib/Logic and Bit Operations/Bit Slice  lidx=MSB  ridx=MSB
      settings: SourceProductBaseCode=SL
  Switch : Switch  Criteria=u2 > Threshold
  Unary Minus : UnaryMinus
  out : Outport
  wires:
  Bit Slice/1 -> Switch/2
  signof/1 -> Bit Slice/1
  base/1 -> Switch/1, Unary Minus/1
  Switch/1 -> out/1
  Unary Minus/1 -> Switch/3

== system kirchImplementation/Filter/CordicAtan/CORDIC Algorithm/Iteration_1/zsign ==
  signof : Inport
  base : Inport  Port=2
  Bit Slice : hdlsllib/Logic and Bit Operations/Bit Slice  lidx=MSB  ridx=MSB
      settings: SourceProductBaseCode=SL
  Switch : Switch  Criteria=u2 > Threshold
  Unary Minus : UnaryMinus
  out : Outport
  wires:
  signof/1 -> Bit Slice/1
  Bit Slice/1 -> Switch/2
  base/1 -> Switch/3, Unary Minus/1
  Switch/1 -> out/1
  Unary Minus/1 -> Switch/1

== system kirchImplementation/Filter/CordicAtan/CORDIC Algorithm/Iteration_10/X_Logic ==
  xo : Inport
  yo : Inport  Port=2
  Add2 : Sum
  Bit Shift : hdlsllib/Logic and Bit Operations/Bit Shift  mode=Shift Right Arithmetic  N=9
  zsign : Subsystem
  x : Outport
  wires:
  yo/1 -> zsign/1(signof), Bit Shift/1
  Bit Shift/1 -> zsign/2(base)
  xo/1 -> Add2/1
  Add2/1 -> x/1
  zsign/1(out) -> Add2/2  "xo"

== system kirchImplementation/Filter/CordicAtan/CORDIC Algorithm/Iteration_10/Y_Logic ==
  xo : Inport
  yo : Inport  Port=2
  Add1 : Sum
  Bit Shift : hdlsllib/Logic and Bit Operations/Bit Shift  mode=Shift Right Arithmetic  N=9
  n_zsign : Subsystem
  y : Outport
  wires:
  Bit Shift/1 -> n_zsign/2(base)
  n_zsign/1(out) -> Add1/2
  Add1/1 -> y/1
  xo/1 -> Bit Shift/1
  yo/1 -> n_zsign/1(signof), Add1/1

== system kirchImplementation/Filter/CordicAtan/CORDIC Algorithm/Iteration_10/n_zsign ==
  signof : Inport
  base : Inport  Port=2
  Bit Slice : hdlsllib/Logic and Bit Operations/Bit Slice  lidx=MSB  ridx=MSB
      settings: SourceProductBaseCode=SL
  Switch : Switch  Criteria=u2 > Threshold
  Unary Minus : UnaryMinus
  out : Outport
  wires:
  Bit Slice/1 -> Switch/2
  signof/1 -> Bit Slice/1
  base/1 -> Switch/1, Unary Minus/1
  Switch/1 -> out/1
  Unary Minus/1 -> Switch/3

== system kirchImplementation/Filter/CordicAtan/CORDIC Algorithm/Iteration_2/X_Logic ==
  xo : Inport
  yo : Inport  Port=2
  Add2 : Sum
  Bit Shift : hdlsllib/Logic and Bit Operations/Bit Shift  mode=Shift Right Arithmetic  N=1
  zsign1 : Subsystem
  x : Outport
  wires:
  yo/1 -> zsign1/1(signof), Bit Shift/1
  Bit Shift/1 -> zsign1/2(base)
  xo/1 -> Add2/1
  Add2/1 -> x/1
  zsign1/1(out) -> Add2/2  "xo"

== system kirchImplementation/Filter/CordicAtan/CORDIC Algorithm/Iteration_2/Y_Logic ==
  xo : Inport
  yo : Inport  Port=2
  Add1 : Sum
  Bit Shift : hdlsllib/Logic and Bit Operations/Bit Shift  mode=Shift Right Arithmetic  N=1
  n_zsign : Subsystem
  y : Outport
  wires:
  Bit Shift/1 -> n_zsign/2(base)
  n_zsign/1(out) -> Add1/2
  Add1/1 -> y/1
  xo/1 -> Bit Shift/1
  yo/1 -> n_zsign/1(signof), Add1/1

== system kirchImplementation/Filter/CordicAtan/CORDIC Algorithm/Iteration_2/n_zsign ==
  signof : Inport
  base : Inport  Port=2
  Bit Slice : hdlsllib/Logic and Bit Operations/Bit Slice  lidx=MSB  ridx=MSB
      settings: SourceProductBaseCode=SL
  Switch : Switch  Criteria=u2 > Threshold
  Unary Minus : UnaryMinus
  out : Outport
  wires:
  Bit Slice/1 -> Switch/2
  signof/1 -> Bit Slice/1
  base/1 -> Switch/1, Unary Minus/1
  Switch/1 -> out/1
  Unary Minus/1 -> Switch/3

== system kirchImplementation/Filter/CordicAtan/CORDIC Algorithm/Iteration_3/X_Logic ==
  xo : Inport
  yo : Inport  Port=2
  Add2 : Sum
  Bit Shift : hdlsllib/Logic and Bit Operations/Bit Shift  mode=Shift Right Arithmetic  N=2
  zsign : Subsystem
  x : Outport
  wires:
  yo/1 -> zsign/1(signof), Bit Shift/1
  Bit Shift/1 -> zsign/2(base)
  xo/1 -> Add2/1
  Add2/1 -> x/1
  zsign/1(out) -> Add2/2  "xo"

== system kirchImplementation/Filter/CordicAtan/CORDIC Algorithm/Iteration_3/Y_Logic ==
  xo : Inport
  yo : Inport  Port=2
  Add1 : Sum
  Bit Shift : hdlsllib/Logic and Bit Operations/Bit Shift  mode=Shift Right Arithmetic  N=2
  n_zsign : Subsystem
  y : Outport
  wires:
  Bit Shift/1 -> n_zsign/2(base)
  n_zsign/1(out) -> Add1/2
  Add1/1 -> y/1
  xo/1 -> Bit Shift/1
  yo/1 -> n_zsign/1(signof), Add1/1

== system kirchImplementation/Filter/CordicAtan/CORDIC Algorithm/Iteration_3/n_zsign ==
  signof : Inport
  base : Inport  Port=2
  Bit Slice : hdlsllib/Logic and Bit Operations/Bit Slice  lidx=MSB  ridx=MSB
      settings: SourceProductBaseCode=SL
  Switch : Switch  Criteria=u2 > Threshold
  Unary Minus : UnaryMinus
  out : Outport
  wires:
  Bit Slice/1 -> Switch/2
  signof/1 -> Bit Slice/1
  base/1 -> Switch/1, Unary Minus/1
  Switch/1 -> out/1
  Unary Minus/1 -> Switch/3

== system kirchImplementation/Filter/CordicAtan/CORDIC Algorithm/Iteration_4/X_Logic ==
  xo : Inport
  yo : Inport  Port=2
  Add2 : Sum
  Bit Shift : hdlsllib/Logic and Bit Operations/Bit Shift  mode=Shift Right Arithmetic  N=3
  zsign : Subsystem
  x : Outport
  wires:
  yo/1 -> zsign/1(signof), Bit Shift/1
  Bit Shift/1 -> zsign/2(base)
  xo/1 -> Add2/1
  Add2/1 -> x/1
  zsign/1(out) -> Add2/2  "xo"

== system kirchImplementation/Filter/CordicAtan/CORDIC Algorithm/Iteration_4/Y_Logic ==
  xo : Inport
  yo : Inport  Port=2
  Add1 : Sum
  Bit Shift : hdlsllib/Logic and Bit Operations/Bit Shift  mode=Shift Right Arithmetic  N=3
  n_zsign : Subsystem
  y : Outport
  wires:
  Bit Shift/1 -> n_zsign/2(base)
  n_zsign/1(out) -> Add1/2
  Add1/1 -> y/1
  xo/1 -> Bit Shift/1
  yo/1 -> n_zsign/1(signof), Add1/1

== system kirchImplementation/Filter/CordicAtan/CORDIC Algorithm/Iteration_4/n_zsign ==
  signof : Inport
  base : Inport  Port=2
  Bit Slice : hdlsllib/Logic and Bit Operations/Bit Slice  lidx=MSB  ridx=MSB
      settings: SourceProductBaseCode=SL
  Switch : Switch  Criteria=u2 > Threshold
  Unary Minus : UnaryMinus
  out : Outport
  wires:
  Bit Slice/1 -> Switch/2
  signof/1 -> Bit Slice/1
  base/1 -> Switch/1, Unary Minus/1
  Switch/1 -> out/1
  Unary Minus/1 -> Switch/3

== system kirchImplementation/Filter/CordicAtan/CORDIC Algorithm/Iteration_5/X_Logic ==
  xo : Inport
  yo : Inport  Port=2
  Add2 : Sum
  Bit Shift : hdlsllib/Logic and Bit Operations/Bit Shift  mode=Shift Right Arithmetic  N=4
  zsign : Subsystem
  x : Outport
  wires:
  yo/1 -> zsign/1(signof), Bit Shift/1
  Bit Shift/1 -> zsign/2(base)
  xo/1 -> Add2/1
  Add2/1 -> x/1
  zsign/1(out) -> Add2/2  "xo"

== system kirchImplementation/Filter/CordicAtan/CORDIC Algorithm/Iteration_5/Y_Logic ==
  xo : Inport
  yo : Inport  Port=2
  Add1 : Sum
  Bit Shift : hdlsllib/Logic and Bit Operations/Bit Shift  mode=Shift Right Arithmetic  N=4
  n_zsign : Subsystem
  y : Outport
  wires:
  Bit Shift/1 -> n_zsign/2(base)
  n_zsign/1(out) -> Add1/2
  Add1/1 -> y/1
  xo/1 -> Bit Shift/1
  yo/1 -> n_zsign/1(signof), Add1/1

== system kirchImplementation/Filter/CordicAtan/CORDIC Algorithm/Iteration_5/n_zsign ==
  signof : Inport
  base : Inport  Port=2
  Bit Slice : hdlsllib/Logic and Bit Operations/Bit Slice  lidx=MSB  ridx=MSB
      settings: SourceProductBaseCode=SL
  Switch : Switch  Criteria=u2 > Threshold
  Unary Minus : UnaryMinus
  out : Outport
  wires:
  Bit Slice/1 -> Switch/2
  signof/1 -> Bit Slice/1
  base/1 -> Switch/1, Unary Minus/1
  Switch/1 -> out/1
  Unary Minus/1 -> Switch/3

== system kirchImplementation/Filter/CordicAtan/CORDIC Algorithm/Iteration_6/X_Logic ==
  xo : Inport
  yo : Inport  Port=2
  Add2 : Sum
  Bit Shift : hdlsllib/Logic and Bit Operations/Bit Shift  mode=Shift Right Arithmetic  N=5
  zsign : Subsystem
  x : Outport
  wires:
  yo/1 -> zsign/1(signof), Bit Shift/1
  Bit Shift/1 -> zsign/2(base)
  xo/1 -> Add2/1
  Add2/1 -> x/1
  zsign/1(out) -> Add2/2  "xo"

== system kirchImplementation/Filter/CordicAtan/CORDIC Algorithm/Iteration_6/Y_Logic ==
  xo : Inport
  yo : Inport  Port=2
  Add1 : Sum
  Bit Shift : hdlsllib/Logic and Bit Operations/Bit Shift  mode=Shift Right Arithmetic  N=5
  n_zsign : Subsystem
  y : Outport
  wires:
  Bit Shift/1 -> n_zsign/2(base)
  n_zsign/1(out) -> Add1/2
  Add1/1 -> y/1
  xo/1 -> Bit Shift/1
  yo/1 -> n_zsign/1(signof), Add1/1

== system kirchImplementation/Filter/CordicAtan/CORDIC Algorithm/Iteration_6/n_zsign ==
  signof : Inport
  base : Inport  Port=2
  Bit Slice : hdlsllib/Logic and Bit Operations/Bit Slice  lidx=MSB  ridx=MSB
      settings: SourceProductBaseCode=SL
  Switch : Switch  Criteria=u2 > Threshold
  Unary Minus : UnaryMinus
  out : Outport
  wires:
  Bit Slice/1 -> Switch/2
  signof/1 -> Bit Slice/1
  base/1 -> Switch/1, Unary Minus/1
  Switch/1 -> out/1
  Unary Minus/1 -> Switch/3
